simulink model "LinearIntegralAntiWindup"  (R2024b)
settings: Solver=FixedStepAuto  StartTime=0  StopTime=120  FixedStep=0.002  RelTol=1e-3
model workspace (MAT data in the model file):
  Disturbance : Simulink.Parameter (value not decoded)
  ToDrvDesigner : Simulink.Parameter (value not decoded)
values from neighbouring files (symbols this model uses):
  C_af = 80000.0    [VehicleData.sldd]
  C_ar = 80000.0    [VehicleData.sldd]
  g = 9.81    [VehicleData.sldd]
  Iz = 2873.0    [VehicleData.sldd]
  lf = 1.1    [VehicleData.sldd]
  lr = 1.58    [VehicleData.sldd]
  m = 2238.932    [VehicleData.sldd]
symbols that are objects in the model workspace (value not decoded): Disturbance
undefined symbols (not defined in the file or in its folder): phi
libraries: slpidlib x9, SignalEditorBlockLib x1
(part 3 of 3)

== matlab function LinearIntegralAntiWindup/LateralController/SMC_ConventionalRegularForm ==
  data: U output size=1; E input; Vx input; dPsi_des input; C_af parameter; g parameter; C_ar parameter; lf parameter; lr parameter; Iz parameter; m parameter; phi_ref input

% ******************* Lateral dynamic controller *********************
%*********************************************************************
% Author: L.Arturo Torres-Romero
% Date: 22-10-2020
% This controller controlls the direction of a car, based in the dynamics
% described  in the next link and using the conventional sliding mode control 
% formulation with the procedure of converting to regular form: 
% https://www.researchgate.net/publication/340166902_LATERAL_VEHICLE_DYNAMICS_AND_CONTROLLERS_DESIGN
%******************* PARAMETERS DESCRIPTIONS **********************
%******************************************************************
% m: vehicle mass
% g: gravity
% C_af : Cornering  stiffness  of  front  wheels.
% C_ar : Cornering  stiffness  of  rear  wheels.
% lf : distance fron the center of gravity to the front wheel axis.
% lr : distance fron the center of gravity to the rear wheel axis.
% Iz : this is the momentum of inertia of the vehicle respect the z axis.
%******************************************************************
%******************* INPUTS DESCRIPTIONS **************************
%******************************************************************
% E:   (column vector)[e1;de1;e2;de2] states of the state space of 
%       the system that includes the errors as follows:
%      e1  : is the lateral position error respect the road.
%      de1 : derivative of e1.
%      e2  : is the yaw angle error with respect the road. 
%      de2 : derivarive of the e2.
% Vx: Logitudinal velocity.

%******************************************************************
% ******************* OUTPUTS DESCRIPTIONS ************************
%******************************************************************
% U: control coutput in radians. Angle of the frontal wheels respect to the
%    longitudinal axis
% isCtrl: when true means that the matrix Mc has full rank, and hence, the
%         system is controllable
%******************************************************************

function U = SMC_ConventionalCtr2(E, Vx, dPsi_des,C_af, g, C_ar, lf, lr, Iz, m, phi_ref) % pd polos deseados
J = [0; 0; 0; 0];
J(1) = E(3);
J(2) = E(4);
J(3) = E(1);
J(4) = E(2);
phi = phi_ref;
%**************************************************
%******* Matrix A formulation *********************
A22 = -(2*C_af + 2*C_ar)/(m*Vx);
A23 = (2*C_af + 2*C_ar)/m;
A24 = (-2*C_af*lf + 2*C_ar*lr)/(m*Vx);
A42 = -(2*C_af*lf - 2*C_ar*lr)/(Iz*Vx);
A43 = (2*C_af*lf - 2*C_ar*lr)/Iz;
A44 = -(2*C_af*lf^2 + 2*C_ar*lr^2)/(Iz*Vx);

%A = [0 1 0 0;0 A22 A23 A24;0 0 0 1;0 A42 A43 A44];
A = [0 0 0 1;0 A42 A43 A44;0 1 0 0;0 A22 A23 A24];

%**************************************************

%**************************************************
%******* Matrix B1 formulation ********************
B1_2 = 2*C_af/m;
B1_4 = 2*C_af*lf/Iz;

%B1 = [0;B1_2;0;B1_4];
B1 = [0;B1_4;0;B1_2];
%***************************************************

%***************************************************
%******* Matrix B2 formulation *********************
B2_2 = -(2*C_af*lf - 2*C_ar*lr)/(m*Vx) - Vx;
B2_4 = -(2*C_af*lf^2 + 2*C_ar*lr^2)/(Iz*Vx);

B2 = [0;B2_4;0;B2_2];
%***************************************************


%***************************************************
%******* Matrix B3 formulation *********************
B3 = [0;g;0;0];
%***************************************************

l1 = (A24 - Vx)*dPsi_des +g*sin(phi);
l2 = A44*dPsi_des;
L = [0;l2;0;l1];

C = [B1 A*B1 A^2*B1 A^3*B1]; % controllability matrix
Cinv = inv(C);
q = Cinv(4,:);
P = [q;q*A;q*A^2;q*A^3];
Tr = P;

X = Tr*J;

%%%%%%%%%%%%%%%%%%%%%%%%%%%%% SMC settings %%%%%%%%%%%%%%%%%%%%%%%%%%%%%%%
n1 = 140000;
lambda_1 = -2;
lambda_2 = -7;
lambda_3 = -3;

S = [(1000000*lambda_1*lambda_2*lambda_3)/(A23*B1_4 - A43*B1_2), (1000000*(A23^2*B1_4^3 + A43^2*B1_2^2*B1_4 + A22*A23*A24*B1_4^3 - A42*A43*A44*B1_2^3 - 2*A23*A43*B1_2*B1_4^2 - A43*A44*B1_2^3*lambda_1 - A43*A44*B1_2^3*lambda_2 - A43*A44*B1_2^3*lambda_3 - A22*A23*A44*B1_2*B1_4^2 - A22*A24*A43*B1_2*B1_4^2 - A23*A24*A42*B1_2*B1_4^2 + A22*A43*A44*B1_2^2*B1_4 + A23*A42*A44*B1_2^2*B1_4 + A24*A42*A43*B1_2^2*B1_4 - A23*A24*B1_2*B1_4^2*lambda_1 - A23*A24*B1_2*B1_4^2*lambda_2 - A23*A24*B1_2*B1_4^2*lambda_3 + A23*A44*B1_2^2*B1_4*lambda_1 + A24*A43*B1_2^2*B1_4*lambda_1 + A23*A44*B1_2^2*B1_4*lambda_2 + A24*A43*B1_2^2*B1_4*lambda_2 + A23*A44*B1_2^2*B1_4*lambda_3 + A24*A43*B1_2^2*B1_4*lambda_3 - A23*B1_2*B1_4^2*lambda_1*lambda_2 - A23*B1_2*B1_4^2*lambda_1*lambda_3 - A23*B1_2*B1_4^2*lambda_2*lambda_3 + A43*B1_2^2*B1_4*lambda_1*lambda_2 + A43*B1_2^2*B1_4*lambda_1*lambda_3 + A43*B1_2^2*B1_4*lambda_2*lambda_3 - A44*B1_2^3*lambda_1*lambda_2*lambda_3 + A22*B1_2*B1_4^2*lambda_1*lambda_2*lambda_3 + A24*B1_2^2*B1_4*lambda_1*lambda_2*lambda_3 - A42*B1_2^2*B1_4*lambda_1*lambda_2*lambda_3))/((A23*B1_4 - A43*B1_2)*(A24^2*B1_2*B1_4^2 - 2*A24*A44*B1_2^2*B1_4 - A42*A24*B1_2*B1_4^2 + A22*A24*B1_4^3 + A44^2*B1_2^3 + A42*A44*B1_2^2*B1_4 - A22*A44*B1_2*B1_4^2 - A43*B1_2*B1_4^2 + A23*B1_4^3)), (1000000*(A23^2*B1_4^3*lambda_1 + A23^2*B1_4^3*lambda_2 + A23^2*B1_4^3*lambda_3 + A23^2*A24*B1_4^3 - A43^2*A44*B1_2^3 + A24*A43^2*B1_2^2*B1_4 - A23^2*A44*B1_2*B1_4^2 + A43^2*B1_2^2*B1_4*lambda_1 + A43^2*B1_2^2*B1_4*lambda_2 + A43^2*B1_2^2*B1_4*lambda_3 - 2*A23*A24*A43*B1_2*B1_4^2 + 2*A23*A43*A44*B1_2^2*B1_4 - 2*A23*A43*B1_2*B1_4^2*lambda_1 - 2*A23*A43*B1_2*B1_4^2*lambda_2 - 2*A23*A43*B1_2*B1_4^2*lambda_3 - A22*A23*B1_4^3*lambda_1*lambda_2 - A22*A23*B1_4^3*lambda_1*lambda_3 - A22*A23*B1_4^3*lambda_2*lambda_3 - A43*A44*B1_2^3*lambda_1*lambda_2 - A43*A44*B1_2^3*lambda_1*lambda_3 - A43*A44*B1_2^3*lambda_2*lambda_3 + A22^2*B1_4^3*lambda_1*lambda_2*lambda_3 + A42^2*B1_2^2*B1_4*lambda_1*lambda_2*lambda_3 - A23*A24*B1_2*B1_4^2*lambda_1*lambda_2 - A23*A24*B1_2*B1_4^2*lambda_1*lambda_3 - A23*A24*B1_2*B1_4^2*lambda_2*lambda_3 + A22*A43*B1_2*B1_4^2*lambda_1*lambda_2 + A23*A42*B1_2*B1_4^2*lambda_1*lambda_2 + A22*A43*B1_2*B1_4^2*lambda_1*lambda_3 + A23*A42*B1_2*B1_4^2*lambda_1*lambda_3 + A22*A43*B1_2*B1_4^2*lambda_2*lambda_3 + A23*A42*B1_2*B1_4^2*lambda_2*lambda_3 + A23*A44*B1_2^2*B1_4*lambda_1*lambda_2 + A24*A43*B1_2^2*B1_4*lambda_1*lambda_2 + A23*A44*B1_2^2*B1_4*lambda_1*lambda_3 + A24*A43*B1_2^2*B1_4*lambda_1*lambda_3 + A23*A44*B1_2^2*B1_4*lambda_2*lambda_3 + A24*A43*B1_2^2*B1_4*lambda_2*lambda_3 - A42*A43*B1_2^2*B1_4*lambda_1*lambda_2 - A42*A43*B1_2^2*B1_4*lambda_1*lambda_3 - A42*A43*B1_2^2*B1_4*lambda_2*lambda_3 + A42*A44*B1_2^3*lambda_1*lambda_2*lambda_3 - A23*B1_2*B1_4^2*lambda_1*lambda_2*lambda_3 + A43*B1_2^2*B1_4*lambda_1*lambda_2*lambda_3 + A22*A24*B1_2*B1_4^2*lambda_1*lambda_2*lambda_3 - 2*A22*A42*B1_2*B1_4^2*lambda_1*lambda_2*lambda_3 - A22*A44*B1_2^2*B1_4*lambda_1*lambda_2*lambda_3 - A24*A42*B1_2^2*B1_4*lambda_1*lambda_2*lambda_3))/((A23*B1_4 - A43*B1_2)*(A24^2*B1_2*B1_4^2 - 2*A24*A44*B1_2^2*B1_4 - A42*A24*B1_2*B1_4^2 + A22*A24*B1_4^3 + A44^2*B1_2^3 + A42*A44*B1_2^2*B1_4 - A22*A44*B1_2*B1_4^2 - A43*B1_2*B1_4^2 + A23*B1_4^3)), (1000000*(A23*A24^2*B1_4^3 - A43*A44^2*B1_2^3 + A23*B1_4^3*lambda_1*lambda_2 + A23*B1_4^3*lambda_1*lambda_3 + A23*B1_4^3*lambda_2*lambda_3 + A23*A44^2*B1_2^2*B1_4 - A24^2*A43*B1_2*B1_4^2 + A23*A24*B1_4^3*lambda_1 + A23*A24*B1_4^3*lambda_2 + A23*A24*B1_4^3*lambda_3 - 2*A23*A24*A44*B1_2*B1_4^2 + 2*A24*A43*A44*B1_2^2*B1_4 - A23*A44*B1_2*B1_4^2*lambda_1 - A24*A43*B1_2*B1_4^2*lambda_1 - A23*A44*B1_2*B1_4^2*lambda_2 - A24*A43*B1_2*B1_4^2*lambda_2 - A23*A44*B1_2*B1_4^2*lambda_3 - A24*A43*B1_2*B1_4^2*lambda_3 + A43*A44*B1_2^2*B1_4*lambda_1 + A43*A44*B1_2^2*B1_4*lambda_2 + A43*A44*B1_2^2*B1_4*lambda_3 - A43*B1_2*B1_4^2*lambda_1*lambda_2 - A43*B1_2*B1_4^2*lambda_1*lambda_3 - A43*B1_2*B1_4^2*lambda_2*lambda_3 - A22*B1_4^3*lambda_1*lambda_2*lambda_3 - A24*B1_2*B1_4^2*lambda_1*lambda_2*lambda_3 + A42*B1_2*B1_4^2*lambda_1*lambda_2*lambda_3 + A44*B1_2^2*B1_4*lambda_1*lambda_2*lambda_3))/((A23*B1_4 - A43*B1_2)*(A24^2*B1_2*B1_4^2 - 2*A24*A44*B1_2^2*B1_4 - A42*A24*B1_2*B1_4^2 + A22*A24*B1_4^3 + A44^2*B1_2^3 + A42*A44*B1_2^2*B1_4 - A22*A44*B1_2*B1_4^2 - A43*B1_2*B1_4^2 + A23*B1_4^3))];

%%%%%%%%%%%%%%%%%%%%%%%%%%%%%%%%%%%%%%%%%%%%%%%%%%%%%%%%%%%%%%%%%%%%%%%%%%%%

sigma1 = S*X;
ctrlVal = -(S*B1)\(n1*sign(sigma1)+ S*A*X +S*L);
U = real(ctrlVal);    



%*****************************************************************************
%******* Live script for help in calculus of the controller ************
% 
% format rational
% syms A B Q R Tr B1_2 B1_4 A22 A23 A24 A42 A43 A44 delta x1 x2 x3 x4 l1 l2
% 
% % X  = [x1;x2;x3;x4]
% % A  = [0 1 0 0;0 A22 A23 A24;0 0 0 1;0 A42 A43 A44]
% % B1 = [0;B1_2;0;B1_4]
% % L  = [0;l1;0;l2]
% 
% X  = [x3;x4;x1;x2]
% A  = [0 0 0 1;0 A42 A43 A44;0 1 0 0;0 A22 A23 A24]
% B1 = [0;B1_4;0;B1_2]
% L  = [0;l2;0;l1]
% 
% %%%%%%%%%%%%%%%% Transform (Tr) with ackerman form %%%%%%%%%%%%%%%%
% % C = [B1 A*B1 A^2*B1 A^3*B1] % controllability matrix
% % tmp1 = [0 0 0 1]/C;
% % Tr=[tmp1;tmp1*A;tmp1*A^2;tmp1*A^3] % state transformation
% % disp("tmp1")
% % size(tmp1)
% % disp("tmp1*A")
% % size(tmp1*A)
% % disp("tmp1*A^2")
% % size(tmp1*A^2)
% % disp("tmp1*A^3")
% % size(tmp1*A^3)
% % disp("C:")
% % size(C)
% % disp("tmp1:")
% % size(tmp1)
% % disp("Tr:")
% % size(Tr)
% %%%%%%%%%%%%%%%%%%%%%%%%%%%%%%%%%%%%%%%%%%%%%%%%%%%%%%%%%%%%%%%%%
% 
% %%%%%%%%%%%% Transform (Tr) with Utkin apprach %%%%%%%%%%%%%%%%%%
% % B_1 = [0;0;B1_4];
% % B_2 = B1_2;
% % 
% % a = eye(3)
% % b = -B_1*(B_2^(-1))
% % c = [0 0 0]
% % d = B_2^(-1)
% % 
% % Tr = [a b;c d];
% %%%%%%%%%%%%%%%%%%%%%%%%%%%%%%%%%%%%%%%%%%%%%%%%%%%%%%%%%%%%%%%%%%
% 
% 
% %%%%%%%%%%%%%%%% Transform (Tr) with linear system controller form %%%%%%%%%%%%%%%%
% C = [B1 A*B1 A^2*B1 A^3*B1] % controllability matrix
% Cinv = inv(C)
% q = Cinv(4,:)
% P = [q;q*A;q*A^2;q*A^3]
% Tr = P
% %%%%%%%%%%%%%%%%%%%%%%%%%%%%%%%%%%%%%%%%%%%%%%%%%%%%%%%%%%
% 
% A_ = simplify(Tr*A/Tr)
% B_ = simplify(Tr*B1)
% 
% A_11 = A_(1:3,1:3);
% A_12 = A_(1:3,4);
% 
% syms s1 s2 s3 lambda lambda_1 lambda_2 lambda_3 S2
% 
% %find paramters given eigenvalues
% S = [s1 s2 s3];
% eqeigen = det(lambda*eye(3) - (A_11 - A_12*S));
% eqeigen = simplify(eqeigen);
% eqeigen = collect(eqeigen,lambda);
% polyCoef = coeffs(eqeigen, lambda);
% polyCoef = fliplr(polyCoef)
% %%%%%%%%%%%%%%%
% % desired polinomial characteristic
% desiredPoly = (lambda + lambda_1)*(lambda + lambda_2)*(lambda + lambda_3);
% desiredPoly = collect(desiredPoly);
% desiredCoefs = coeffs(desiredPoly, lambda);
% desiredCoefs = fliplr(desiredCoefs)
% 
% eq1 = desiredCoefs(1) == polyCoef(1);
% eq2 = desiredCoefs(2) == polyCoef(2);
% eq3 = desiredCoefs(3) == polyCoef(3);
% eq4 = desiredCoefs(4) == polyCoef(4);
% 
% system1 = [eq2;eq3;eq4];
% sol = solve(system1,[s1 s2 s3]);
% S_ = [sol.s1 sol.s2 sol.s3]
% 
% %test eigen values:
% charEq1 = subs(eqeigen,s1,sol.s1);
% charEq2 = subs(charEq1,s2,sol.s2);
% charEq3 = subs(charEq2,s3,sol.s3)
% tf = isAlways(charEq3==desiredPoly)
% 
% S2 = 1000000;
% S = S2*[S_ 1]*Tr;
% %S = [S_ 1]*Tr;
% disp("!!!!!!!!surface S: ")
% simplify(S)
% 
% 
% syms n sigma1 x1 x2 x3 x4 u1 u2 n1 n2 
% X = [x1;x2;x3;x4];
% U = u1;
% 
% SIGMA = S*X;
% 
% % rewriting to the original forms %%%%%%%%%%%%%%%
% X  = [x1;x2;x3;x4]
% A  = [0 1 0 0;0 A22 A23 A24;0 0 0 1;0 A42 A43 A44]
% B1 = [0;B1_2;0;B1_4]
% %%%%%%%%%%%%%%%%%%%%%%%%%%%%%%%%%%%%%%%%%%%%%%%
% 
% 
% disp("!!!!! Sliding function sigma_1: ")
% Sigma_1 = simplify(SIGMA);
% Sigma_1 = collect(Sigma_1,[x1;x2;x3;x4])
% 
% eqsolution = -n1*sign(sigma1) == S*(A*X + B1*U +L);
% sol1 = solve(eqsolution,u1);
% 
% disp("!!!!! final control u: ")
% finalControl = simplify(sol1);
% finalControl = collect(finalControl,[x1;x2;x3;x4])
% 
% 
% U = -inv(S*B1)*(n1*sign(sigma1)+ S*A*X +S*L)
% 
% isAlways(finalControl==U)

== matlab function LinearIntegralAntiWindup/LateralController/HOSMC_IntegralBlocksSuperTwisting/HOSMC_SuperTwisting ==
  data: U output size=1; E input; Vx input; dPsi_des input; phi_ref input; v input; Y1n input; Y2n input; C_af parameter; g parameter; C_ar parameter; lf parameter; lr parameter; Iz parameter; m parameter; dv output; d_u output; dY1n output; dY2n output
% ******************* Lateral dynamic controller *********************

%*********************************************************************
% Author: L.Arturo Torres-Romero
% Date: 22-10-2020
% This controller controlls the direction of a car, based in the dynamics
% described  in the next link and using the conventional sliding mode control 
% formulation with the procedure of converting to regular form: 
% https://www.researchgate.net/publication/340166902_LATERAL_VEHICLE_DYNAMICS_AND_CONTROLLERS_DESIGN
%******************* PARAMETERS DESCRIPTIONS **********************
%******************************************************************
% m: vehicle mass
% g: gravity
% C_af : Cornering  stiffness  of  front  wheels.
% C_ar : Cornering  stiffness  of  rear  wheels.
% lf : distance fron the center of gravity to the front wheel axis.
% lr : distance fron the center of gravity to the rear wheel axis.
% Iz : this is the momentum of inertia of the vehicle respect the z axis.
%******************************************************************
%******************* INPUTS DESCRIPTIONS **************************
%******************************************************************
% E:   (column vector)[e1;de1;e2;de2] states of the state space of 
%       the system that includes the errors as follows:
%      e1  : is the lateral position error respect the road.
%      de1 : derivative of e1.
%      e2  : is the yaw angle error with respect the road. 
%      de2 : derivarive of the e2.
% Vx: Logitudinal velocity.

%******************************************************************
% ******************* OUTPUTS DESCRIPTIONS ************************
%******************************************************************
% U: control coutput in radians. Angle of the frontal wheels respect to the
%    longitudinal axis
% isCtrl: when true means that the matrix Mc has full rank, and hence, the
%         system is controllable
%******************************************************************

function [U, dv,d_u,dY1n,dY2n] = HOSMC_SuperTwistingCtrl(E, Vx,dPsi_des, phi_ref, v,Y1n, Y2n, C_af, g, C_ar, lf, lr, Iz, m) % pd polos deseados
Y1 = [0;0];
Y2 = [0;0];

Y1 = [E(1);E(3)];
Y2 = [E(2);E(4)];
e = [E(2);E(3);E(4)];
en = [Y2n(1); Y1n(2); Y2n(2)];
phi = phi_ref;

%**************************************************
%******* Matrix A formulation *********************
A22 = -(2*C_af + 2*C_ar)/(m*Vx);
A23 = (2*C_af + 2*C_ar)/m;
A24 = (-2*C_af*lf + 2*C_ar*lr)/(m*Vx);
A42 = -(2*C_af*lf - 2*C_ar*lr)/(Iz*Vx);
A43 = (2*C_af*lf - 2*C_ar*lr)/Iz;
A44 = -(2*C_af*lf^2 + 2*C_ar*lr^2)/(Iz*Vx);

A = [A22 A23 A24;A42 A43 A44];

%**************************************************
%******* Matrix B1 formulation ********************
B1_2 = 2*C_af/m;
B1_4 = 2*C_af*lf/Iz;

B1 = [B1_2;B1_4];
%***************************************************

%***************************************************
%******* Matrix L formulation *********************
l1 = (A24 - Vx)*dPsi_des +g*sin(phi);
l2 = A44*dPsi_des;
L = [l1;l2];

%***************************************************

%%
%%%%%%%%%%%%%% SUPER TWISTING 1 %%%%%%%%%%%%%%%%%
% %*********** Controller parameters **************
% k1 = 1;%6;      %7   18
% k2 = 15;%8;
%sigma = 10;    %60   10
gamma1 = 10;
gamma2 = 1;
gamma = [gamma1 gamma2];
%***************************************
h_c = abs(gamma*[0.8;0.4]);
g_c = abs(gamma*B1);
U_M = pi/16;

q = abs(h_c/g_c)/U_M + 0.01;
C = abs(h_c)+ 0.3;
k_v = C/(gamma*B1) + 0.2; %k_v = C/(gamma*B1) + 0.5;

k_u = sqrt(2/(gamma*B1*k_v - C));
k_u = k_u*(gamma*B1*k_v + C)*(1+q);
k_u = k_u/((gamma*B1)*(1-q)) + 0.1; %k_u = k_u/((gamma*B1)*(1-q)) + 0.8;

k_v = k_v+2;
k_u = k_u+0.1;

%***********************************************
k1 = 36;%6;      %7   18
k2 = 8;%8;
e_b = -gamma*(k1*Y1+Y2);
d_k = -(1/(gamma*B1))*(gamma*(k1*Y2+A*e+L)-k2*e_b);


dY2n = A*e + B1*d_k + L;
dY1n = Y2n;

e_t = gamma*(Y1+Y2);
e_tn = gamma*(Y1n+Y2n);

%Y2_0 = [0; 21.15];
%Y2_0 = [0; 0];

s = e_t - e_tn;

d_u = -k_u*sqrt(abs(s))*sign(s) + v;

if abs(d_u) > U_M 
   dv = -d_u;
else
   dv = -k_v*sign(s); 
end

%%

ctrlVal = d_k;
ctrlVal = d_k + d_u;
U = real(ctrlVal);

== matlab function LinearIntegralAntiWindup/LateralController/HOSMC_RegularFormSuperTwist/HOSMC_RegularFormSuperTwist ==
  data: U output size=1; E input; Vx input; dPsi_des input; Mu1 input; C_af parameter; g parameter; C_ar parameter; lf parameter; lr parameter; Iz parameter; m parameter; dMu1 output; phi parameter
% ******************* Lateral dynamic controller *********************

%*********************************************************************
% Author: L.Arturo Torres-Romero
% Date: 22-10-2020
% This controller controlls the direction of a car, based in the dynamics
% described  in the next link and using the conventional sliding mode control 
% formulation with the procedure of converting to regular form: 
% https://www.researchgate.net/publication/340166902_LATERAL_VEHICLE_DYNAMICS_AND_CONTROLLERS_DESIGN
%******************* PARAMETERS DESCRIPTIONS **********************
%******************************************************************
% m: vehicle mass
% g: gravity
% C_af : Cornering  stiffness  of  front  wheels.
% C_ar : Cornering  stiffness  of  rear  wheels.
% lf : distance fron the center of gravity to the front wheel axis.
% lr : distance fron the center of gravity to the rear wheel axis.
% Iz : this is the momentum of inertia of the vehicle respect the z axis.
%******************************************************************
%******************* INPUTS DESCRIPTIONS **************************
%******************************************************************
% E:   (column vector)[e1;de1;e2;de2] states of the state space of 
%       the system that includes the errors as follows:
%      e1  : is the lateral position error respect the road.
%      de1 : derivative of e1.
%      e2  : is the yaw angle error with respect the road. 
%      de2 : derivarive of the e2.
% Vx: Logitudinal velocity.

%******************************************************************
% ******************* OUTPUTS DESCRIPTIONS ************************
%******************************************************************
% U: control coutput in radians. Angle of the frontal wheels respect to the
%    longitudinal axis
% isCtrl: when true means that the matrix Mc has full rank, and hence, the
%         system is controllable
%******************************************************************

function [U, dMu1] = HOSMC_RegularFormSuperTwistCtrl(E, Vx,dPsi_des, Mu1,C_af, g, C_ar, lf, lr, Iz, m,phi) % pd polos deseados
J = [0; 0; 0; 0];
J(1) = E(3);
J(2) = E(4);
J(3) = E(1);
J(4) = E(2);

%**************************************************
%******* Matrix A formulation *********************
A22 = -(2*C_af + 2*C_ar)/(m*Vx);
A23 = (2*C_af + 2*C_ar)/m;
A24 = (-2*C_af*lf + 2*C_ar*lr)/(m*Vx);
A42 = -(2*C_af*lf - 2*C_ar*lr)/(Iz*Vx);
A43 = (2*C_af*lf - 2*C_ar*lr)/Iz;
A44 = -(2*C_af*lf^2 + 2*C_ar*lr^2)/(Iz*Vx);

%A = [0 1 0 0;0 A22 A23 A24;0 0 0 1;0 A42 A43 A44];
A = [0 0 0 1;0 A42 A43 A44;0 1 0 0;0 A22 A23 A24];

%**************************************************

%**************************************************
%******* Matrix B1 formulation ********************
B1_2 = 2*C_af/m;
B1_4 = 2*C_af*lf/Iz;

%B1 = [0;B1_2;0;B1_4];
B1 = [0;B1_4;0;B1_2];
%***************************************************

%***************************************************
%******* Matrix B2 formulation *********************
B2_2 = -(2*C_af*lf - 2*C_ar*lr)/(m*Vx) - Vx;
B2_4 = -(2*C_af*lf^2 + 2*C_ar*lr^2)/(Iz*Vx);

B2 = [0;B2_4;0;B2_2];
%***************************************************


%***************************************************
%******* Matrix B3 formulation *********************
B3 = [0;g;0;0];
%***************************************************

l1 = (A24 - Vx)*dPsi_des +g*sin(phi);
l2 = A44*dPsi_des;
L = [0;l2;0;l1];

C = [B1 A*B1 A^2*B1 A^3*B1]; % controllability matrix
Cinv = inv(C);
q = Cinv(4,:);
P = [q;q*A;q*A^2;q*A^3];
Tr = P;

X = Tr*J;

%%%%%%%%%%%%%%%%%%%%%%%%%%%%% SMC settings %%%%%%%%%%%%%%%%%%%%%%%%%%%%%%%
n1 = 1;%140000;
lambda_1 = -2;
lambda_2 = -7;
lambda_3 = -3;

S = [(1000000*lambda_1*lambda_2*lambda_3)/(A23*B1_4 - A43*B1_2), (1000000*(A23^2*B1_4^3 + A43^2*B1_2^2*B1_4 + A22*A23*A24*B1_4^3 - A42*A43*A44*B1_2^3 - 2*A23*A43*B1_2*B1_4^2 - A43*A44*B1_2^3*lambda_1 - A43*A44*B1_2^3*lambda_2 - A43*A44*B1_2^3*lambda_3 - A22*A23*A44*B1_2*B1_4^2 - A22*A24*A43*B1_2*B1_4^2 - A23*A24*A42*B1_2*B1_4^2 + A22*A43*A44*B1_2^2*B1_4 + A23*A42*A44*B1_2^2*B1_4 + A24*A42*A43*B1_2^2*B1_4 - A23*A24*B1_2*B1_4^2*lambda_1 - A23*A24*B1_2*B1_4^2*lambda_2 - A23*A24*B1_2*B1_4^2*lambda_3 + A23*A44*B1_2^2*B1_4*lambda_1 + A24*A43*B1_2^2*B1_4*lambda_1 + A23*A44*B1_2^2*B1_4*lambda_2 + A24*A43*B1_2^2*B1_4*lambda_2 + A23*A44*B1_2^2*B1_4*lambda_3 + A24*A43*B1_2^2*B1_4*lambda_3 - A23*B1_2*B1_4^2*lambda_1*lambda_2 - A23*B1_2*B1_4^2*lambda_1*lambda_3 - A23*B1_2*B1_4^2*lambda_2*lambda_3 + A43*B1_2^2*B1_4*lambda_1*lambda_2 + A43*B1_2^2*B1_4*lambda_1*lambda_3 + A43*B1_2^2*B1_4*lambda_2*lambda_3 - A44*B1_2^3*lambda_1*lambda_2*lambda_3 + A22*B1_2*B1_4^2*lambda_1*lambda_2*lambda_3 + A24*B1_2^2*B1_4*lambda_1*lambda_2*lambda_3 - A42*B1_2^2*B1_4*lambda_1*lambda_2*lambda_3))/((A23*B1_4 - A43*B1_2)*(A24^2*B1_2*B1_4^2 - 2*A24*A44*B1_2^2*B1_4 - A42*A24*B1_2*B1_4^2 + A22*A24*B1_4^3 + A44^2*B1_2^3 + A42*A44*B1_2^2*B1_4 - A22*A44*B1_2*B1_4^2 - A43*B1_2*B1_4^2 + A23*B1_4^3)), (1000000*(A23^2*B1_4^3*lambda_1 + A23^2*B1_4^3*lambda_2 + A23^2*B1_4^3*lambda_3 + A23^2*A24*B1_4^3 - A43^2*A44*B1_2^3 + A24*A43^2*B1_2^2*B1_4 - A23^2*A44*B1_2*B1_4^2 + A43^2*B1_2^2*B1_4*lambda_1 + A43^2*B1_2^2*B1_4*lambda_2 + A43^2*B1_2^2*B1_4*lambda_3 - 2*A23*A24*A43*B1_2*B1_4^2 + 2*A23*A43*A44*B1_2^2*B1_4 - 2*A23*A43*B1_2*B1_4^2*lambda_1 - 2*A23*A43*B1_2*B1_4^2*lambda_2 - 2*A23*A43*B1_2*B1_4^2*lambda_3 - A22*A23*B1_4^3*lambda_1*lambda_2 - A22*A23*B1_4^3*lambda_1*lambda_3 - A22*A23*B1_4^3*lambda_2*lambda_3 - A43*A44*B1_2^3*lambda_1*lambda_2 - A43*A44*B1_2^3*lambda_1*lambda_3 - A43*A44*B1_2^3*lambda_2*lambda_3 + A22^2*B1_4^3*lambda_1*lambda_2*lambda_3 + A42^2*B1_2^2*B1_4*lambda_1*lambda_2*lambda_3 - A23*A24*B1_2*B1_4^2*lambda_1*lambda_2 - A23*A24*B1_2*B1_4^2*lambda_1*lambda_3 - A23*A24*B1_2*B1_4^2*lambda_2*lambda_3 + A22*A43*B1_2*B1_4^2*lambda_1*lambda_2 + A23*A42*B1_2*B1_4^2*lambda_1*lambda_2 + A22*A43*B1_2*B1_4^2*lambda_1*lambda_3 + A23*A42*B1_2*B1_4^2*lambda_1*lambda_3 + A22*A43*B1_2*B1_4^2*lambda_2*lambda_3 + A23*A42*B1_2*B1_4^2*lambda_2*lambda_3 + A23*A44*B1_2^2*B1_4*lambda_1*lambda_2 + A24*A43*B1_2^2*B1_4*lambda_1*lambda_2 + A23*A44*B1_2^2*B1_4*lambda_1*lambda_3 + A24*A43*B1_2^2*B1_4*lambda_1*lambda_3 + A23*A44*B1_2^2*B1_4*lambda_2*lambda_3 + A24*A43*B1_2^2*B1_4*lambda_2*lambda_3 - A42*A43*B1_2^2*B1_4*lambda_1*lambda_2 - A42*A43*B1_2^2*B1_4*lambda_1*lambda_3 - A42*A43*B1_2^2*B1_4*lambda_2*lambda_3 + A42*A44*B1_2^3*lambda_1*lambda_2*lambda_3 - A23*B1_2*B1_4^2*lambda_1*lambda_2*lambda_3 + A43*B1_2^2*B1_4*lambda_1*lambda_2*lambda_3 + A22*A24*B1_2*B1_4^2*lambda_1*lambda_2*lambda_3 - 2*A22*A42*B1_2*B1_4^2*lambda_1*lambda_2*lambda_3 - A22*A44*B1_2^2*B1_4*lambda_1*lambda_2*lambda_3 - A24*A42*B1_2^2*B1_4*lambda_1*lambda_2*lambda_3))/((A23*B1_4 - A43*B1_2)*(A24^2*B1_2*B1_4^2 - 2*A24*A44*B1_2^2*B1_4 - A42*A24*B1_2*B1_4^2 + A22*A24*B1_4^3 + A44^2*B1_2^3 + A42*A44*B1_2^2*B1_4 - A22*A44*B1_2*B1_4^2 - A43*B1_2*B1_4^2 + A23*B1_4^3)), (1000000*(A23*A24^2*B1_4^3 - A43*A44^2*B1_2^3 + A23*B1_4^3*lambda_1*lambda_2 + A23*B1_4^3*lambda_1*lambda_3 + A23*B1_4^3*lambda_2*lambda_3 + A23*A44^2*B1_2^2*B1_4 - A24^2*A43*B1_2*B1_4^2 + A23*A24*B1_4^3*lambda_1 + A23*A24*B1_4^3*lambda_2 + A23*A24*B1_4^3*lambda_3 - 2*A23*A24*A44*B1_2*B1_4^2 + 2*A24*A43*A44*B1_2^2*B1_4 - A23*A44*B1_2*B1_4^2*lambda_1 - A24*A43*B1_2*B1_4^2*lambda_1 - A23*A44*B1_2*B1_4^2*lambda_2 - A24*A43*B1_2*B1_4^2*lambda_2 - A23*A44*B1_2*B1_4^2*lambda_3 - A24*A43*B1_2*B1_4^2*lambda_3 + A43*A44*B1_2^2*B1_4*lambda_1 + A43*A44*B1_2^2*B1_4*lambda_2 + A43*A44*B1_2^2*B1_4*lambda_3 - A43*B1_2*B1_4^2*lambda_1*lambda_2 - A43*B1_2*B1_4^2*lambda_1*lambda_3 - A43*B1_2*B1_4^2*lambda_2*lambda_3 - A22*B1_4^3*lambda_1*lambda_2*lambda_3 - A24*B1_2*B1_4^2*lambda_1*lambda_2*lambda_3 + A42*B1_2*B1_4^2*lambda_1*lambda_2*lambda_3 + A44*B1_2^2*B1_4*lambda_1*lambda_2*lambda_3))/((A23*B1_4 - A43*B1_2)*(A24^2*B1_2*B1_4^2 - 2*A24*A44*B1_2^2*B1_4 - A42*A24*B1_2*B1_4^2 + A22*A24*B1_4^3 + A44^2*B1_2^3 + A42*A44*B1_2^2*B1_4 - A22*A44*B1_2*B1_4^2 - A43*B1_2*B1_4^2 + A23*B1_4^3))];

%%%%%%%%%%%%%%%%%%%%%%%%%%%%%%%%%%%%%%%%%%%%%%%%%%%%%%%%%%%%%%%%%%%%%%%%%%%%

k_smc = 1000*1.5;   %10
sigma = 6000*1.5;    %60

sigma1 = S*X;

d_k = -(S*B1)\(S*A*X +S*L);
d_u = -(S*B1)\(n1*sigma*sqrt(abs(sigma1))*sign(sigma1) + Mu1);
dMu1 = -k_smc*sign(sigma1); 

ctrlVal = d_k + d_u;
U = real(ctrlVal);

== matlab function LinearIntegralAntiWindup/SteerActuator/BLDC_AngleCtrl/Back EMF ==
  data: X input; Fabc output
function Fabc = fcn(X)
Fabc = [0;0;0];
    theta = mod(X(5),2*pi); %X(4)
    %theta = mod(X,2*pi);
    
    if (0<=theta)&&(theta<(pi/6))
        Fa = (6/pi)*theta;
    elseif ((pi/6)<=theta)&&(theta<(5*pi/6))
        Fa = 1;
    elseif ((5*pi/6<=theta))&&(theta<(7*pi/6))
        Fa = (6/pi)*(pi-theta);
    elseif ((7*pi/6)<=theta)&&(theta<(11*pi/6))
        Fa = -1;
    elseif ((11*pi/6)<=theta)&&(theta<(2*pi))
        Fa = (6/pi)*(theta-2*pi);
    else
        Fa = NaN;
    end
    
    if (0<=theta)&&(theta<(3*pi/6))
        Fb = -1;
    elseif ((3*pi/6)<=theta)&&(theta<(5*pi/6))
        Fb = (6/pi)*(theta-(2*pi)/3);
    elseif ((5*pi/6)<=theta)&&(theta<(9*pi/6))
        Fb = 1;
    elseif ((9*pi/6)<=theta)&&(theta<(11*pi/6))
        Fb = (6/pi)*(-theta+(5*pi)/3);
    elseif ((11*pi/6)<=theta)&&(theta<(2*pi))
        Fb = -1;
    else
        Fb = NaN;
    end
    
    if (0<=theta)&&(theta<(pi/6))
        Fc = 1;
    elseif ((pi/6)<=theta)&&(theta<(3*pi/6))
        Fc = (6/pi)*(pi/3-theta);
    elseif ((3*pi/6)<=theta)&&(theta<(7*pi/6))
        Fc = -1;
    elseif ((7*pi/6)<=theta)&&(theta<(9*pi/6))
        Fc = (6/pi)*(theta-(4*pi)/3);
    elseif ((9*pi/6)<=theta)&&(theta<(2*pi))
        Fc = 1;
    else
        Fc = NaN; 
    end
    
    
%     
     %Fa = sin(theta);
     %Fb = sin(theta - 2*pi/3);
     %Fc = sin(theta + 2*pi/3);
    
    Fabc = [Fa;Fb;Fc];
end

== matlab function LinearIntegralAntiWindup/SteerActuator/BLDC_AngleCtrl/InvParkClarke ==
  data: X_dq input; Y_abc output; theta input
function Y_abc = fcn(X_dq, theta)
X_dq0 = [X_dq; 0];

%inverse Park-Clarke power invariant
iT_PC = sqrt(2/3)*[cos(theta)          -sin(theta)            1/sqrt(2); ...
                  cos(theta-2*pi/3)   -sin(theta-2*pi/3)     1/sqrt(2); ...
                  cos(theta+2*pi/3)   -sin(theta+2*pi/3)     1/sqrt(2)];
%               
              
 %inverse Park-Clarke amplitude invariant
% iT_PC = [cos(theta)          -sin(theta)            1; ...
%          cos(theta-2*pi/3)   -sin(theta-2*pi/3)     1; ...
%          cos(theta+2*pi/3)   -sin(theta+2*pi/3)     1];



Y_abc =iT_PC*X_dq0;
end

== matlab function LinearIntegralAntiWindup/MATLAB Function2 ==
  settings: updateMethod=DISCRETE
  data: u input; maxVal output; meanVal output
function [maxVal, meanVal] = statsSignal(u)
%#codegen

% Variables persistentes para acumular datos
persistent max_so_far sum_so_far count_so_far

if isempty(max_so_far)
    max_so_far  = -inf;   % Valor inicial muy bajo
    sum_so_far  = 0;
    count_so_far = 0;
end

% Actualizar máximo
if u > max_so_far
    max_so_far = u;
end

% Acumular para promedio
sum_so_far = sum_so_far + u;
count_so_far = count_so_far + 1;

% Calcular promedio
meanVal = sum_so_far / count_so_far;

% Salida de máximo
maxVal = max_so_far;

== matlab function LinearIntegralAntiWindup/SteerActuator/BLDC_AngleCtrl/ParkClarke ==
  data: X_abc input; Y_dq output; theta input
function Y_dq = fcn(X_abc, theta)

% Park clarke transform eliminating the third element
PC_T = (sqrt(2)/2)*[sqrt(3)*cos(theta)  sin(theta)  -sin(theta) ; ...
                    -sqrt(3)*sin(theta)  cos(theta)  -cos(theta)];

Y_dq =PC_T*X_abc;
end

== matlab function LinearIntegralAntiWindup/LateralController/HOSMC_IntegralNestedST/HOSMC_SuperTwisting ==
  data: U output size=1; dY2n output; E input; Vx input; dPsi_des input; phi_ref input; Y2n input; mu2 input; C_af parameter; g parameter; C_ar parameter; lf parameter; lr parameter; Iz parameter; m parameter; dmu2 output
% ******************* Lateral dynamic controller *********************

%*********************************************************************
% Author: L.Arturo Torres-Romero
% Date: 22-10-2020
% This controller controlls the direction of a car, based in the dynamics
% described  in the next link and using the conventional sliding mode control 
% formulation with the procedure of converting to regular form: 
% https://www.researchgate.net/publication/340166902_LATERAL_VEHICLE_DYNAMICS_AND_CONTROLLERS_DESIGN
%******************* PARAMETERS DESCRIPTIONS **********************
%******************************************************************
% m: vehicle mass
% g: gravity
% C_af : Cornering  stiffness  of  front  wheels.
% C_ar : Cornering  stiffness  of  rear  wheels.
% lf : distance fron the center of gravity to the front wheel axis.
% lr : distance fron the center of gravity to the rear wheel axis.
% Iz : this is the momentum of inertia of the vehicle respect the z axis.
%******************************************************************
%******************* INPUTS DESCRIPTIONS **************************
%******************************************************************
% E:   (column vector)[e1;de1;e2;de2] states of the state space of 
%       the system that includes the errors as follows:
%      e1  : is the lateral position error respect the road.
%      de1 : derivative of e1.
%      e2  : is the yaw angle error with respect the road. 
%      de2 : derivarive of the e2.
% Vx: Logitudinal velocity.

%******************************************************************
% ******************* OUTPUTS DESCRIPTIONS ************************
%******************************************************************
% U: control coutput in radians. Angle of the frontal wheels respect to the
%    longitudinal axis
% isCtrl: when true means that the matrix Mc has full rank, and hence, the
%         system is controllable
%******************************************************************

function [U,dY2n,dmu2] = HOSMC_SuperTwistingCtrl(E, Vx,dPsi_des, phi_ref,Y2n,mu2,C_af, g, C_ar, lf, lr, Iz, m) % pd polos deseados
%function U  = HOSMC_SuperTwistingCtrl(E, Vx,dPsi_des, phi_ref, C_af, g, C_ar, lf, lr, Iz, m) % pd polos deseados
Y1 = [0;0];
Y2 = [0;0];
dY2n = [0;0];

Y1 = [E(1);E(3)];
Y2 = [E(2);E(4)];
e = [E(2);E(3);E(4)]; 
phi = phi_ref;


%**************************************************
%******* Matrix A formulation *********************
A22 = -(2*C_af + 2*C_ar)/(m*Vx);
A23 = (2*C_af + 2*C_ar)/m;
A24 = (-2*C_af*lf + 2*C_ar*lr)/(m*Vx);
A42 = -(2*C_af*lf - 2*C_ar*lr)/(Iz*Vx);
A43 = (2*C_af*lf - 2*C_ar*lr)/Iz;
A44 = -(2*C_af*lf^2 + 2*C_ar*lr^2)/(Iz*Vx);

A = [A22 A23 A24;A42 A43 A44];

%**************************************************
%******* Matrix B1 formulation ********************
B1_2 = 2*C_af/m;
B1_4 = 2*C_af*lf/Iz;

B1 = [B1_2;B1_4];
%***************************************************

%***************************************************
%******* Matrix L formulation *********************
l1 = (A24 - Vx)*dPsi_des +g*sin(phi);
l2 = A44*dPsi_des;
L = [l1;l2];

%***************************************************

%% Nominal control and response

%***********************************************
gamma1 = 1;
gamma2 = 1;
gamma = [gamma1 gamma2];

se1 = gamma*Y1;
se2 = gamma*Y2;

epsilon = 20;
sigma1 = 0.1;
k1=2;

% se2ref = -sigma1*sqrt(abs(se1))*tanh(epsilon*se1)+mu1;
% dmu1 = -k1*sign(se1);

dse2ref = f_dSTA (se1,sigma1,k1,epsilon);

d_k = (1/(gamma*B1))*(dse2ref - gamma*(A*e + L));
%***************************************************************
%% Control for disturbances

se2_0 = 0;
dY2n = A*e + L + B1*d_k;
se2n = gamma*Y2n;
se4 = (se2-se2n);

sigma2 = 0.1; %0.5
k2=0.8;      %1
d_u = -sigma2*sqrt(abs(se4))*sign(se4) + mu2;
dmu2 = -k2*sign(se4);


% %........................................................................
%%

%ctrlVal = d_k;
ctrlVal = d_k + d_u;
U = real(ctrlVal);    

end




function y = f_dSTA (x,sigma,k,epsilon)
    
    t = (abs(x))^(-1/2); 
    if isinf(t)
        t = 10000;
    elseif t >10000
        t = 10000;
    end
    
    y = -sigma*(1/2)*t*tanh(epsilon*x)*sign(x) ...
        -epsilon*sigma*sqrt(abs(x))*(1 - tanh(epsilon*x)^2)...
        -k*sign(x);
end


function y = sat_d (x,max_d_u)
    y = x;
    if x > max_d_u
        y = max_d_u;
    elseif x < -max_d_u
        y = -max_d_u;
    end
end

== matlab function LinearIntegralAntiWindup/MATLAB Function ==
  data: E input; dd input; dE output; Vx input; dPsi_des input; phi_ref input; NoiseDdy input; NoiseDdpsi input; Iz parameter; m parameter; lr parameter; lf parameter; C_ar parameter; g parameter; C_af parameter
function dE = HOSMC_SuperTwistingCtrl(E, dd,Vx,dPsi_des, phi_ref, NoiseDdy, NoiseDdpsi, Iz, m, lr, lf, C_ar, g, C_af) % pd polos deseados
phi = phi_ref;

%**************************************************
%******* Matrix A formulation *********************
A22 = -(2*C_af + 2*C_ar)/(m*Vx);
A23 = (2*C_af + 2*C_ar)/m;
A24 = (-2*C_af*lf + 2*C_ar*lr)/(m*Vx);
A42 = -(2*C_af*lf - 2*C_ar*lr)/(Iz*Vx);
A43 = (2*C_af*lf - 2*C_ar*lr)/Iz;
A44 = -(2*C_af*lf^2 + 2*C_ar*lr^2)/(Iz*Vx);

A = [0 1 0 0;0 A22 A23 A24;0 0 0 1;0 A42 A43 A44];

%**************************************************
%******* Matrix B1 formulation ********************
B1_2 = 2*C_af/m;
B1_4 = 2*C_af*lf/Iz;

B1 = [0; B1_2; 0; B1_4];
%***************************************************

%***************************************************
%******* Matrix L formulation *********************
l1 = (A24 - Vx)*dPsi_des +g*sin(phi);
l2 = A44*dPsi_des;
L = [0; l1;0; l2];

disturbance = [0;NoiseDdy;0; NoiseDdpsi];

%***************************************************

dE = A*E + B1.*dd + L +disturbance;

== matlab function LinearIntegralAntiWindup/LateralController/HOSMC_IntegralBlocksSuperTwisting/MATLAB Function2 ==
  data: u input; y output
function y = fcn(u)
L = pi/8;
e = 1;

y = L.*tanh(u./e);
